simulink model "linear_bounded"  (R2017b)
settings: Solver=VariableStepAuto  StartTime=0.0  StopTime=1000  FixedStep=10e-3
settings Model: Creator=Mehmet  LastModifiedBy=Mehmet

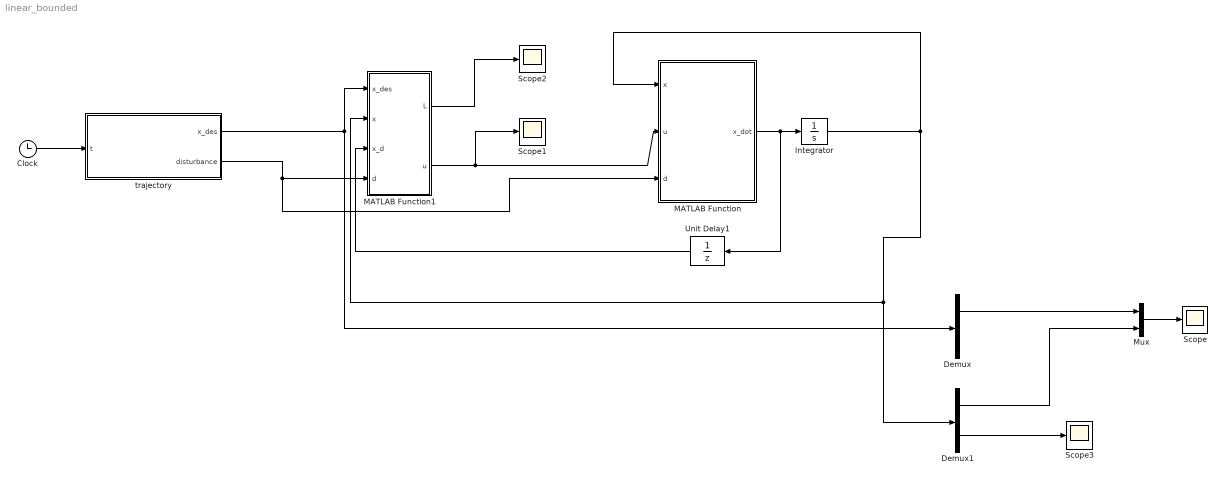
== system linear_bounded ==
  Clock : Clock
  Demux : Demux  Outputs=2
  Demux1 : Demux  Outputs=2
  Integrator : Integrator  InitialCondition=[1;-1]
  MATLAB Function : MATLAB Function  TreatAsAtomicUnit=on
  MATLAB Function1 : MATLAB Function  TreatAsAtomicUnit=on
  Mux : Mux  Inputs=2
  Scope{,1..3} (4 alike) : Scope
  Unit Delay1 : UnitDelay  SampleTime=-1
  trajectory : MATLAB Function  TreatAsAtomicUnit=on
  wires:
  Clock/1 -> trajectory/1(t)
  trajectory/1(x_des) -> MATLAB Function1/1(x_des), Demux/1
  Mux/1 -> Scope/1
  MATLAB Function/1(x_dot) -> Unit Delay1/1, Integrator/1
  Integrator/1 -> Demux1/1, MATLAB Function1/2(x), MATLAB Function/1(x)
  Unit Delay1/1 -> MATLAB Function1/3(x_d)
  trajectory/2(disturbance) -> MATLAB Function1/4(d), MATLAB Function/3(d)
  MATLAB Function1/2(u) -> Scope1/1, MATLAB Function/2(u)
  MATLAB Function1/1(L) -> Scope2/1
  Demux/1 -> Mux/1
  Demux1/1 -> Mux/2
  Demux1/2 -> Scope3/1

== matlab function linear_bounded/MATLAB Function1 ==
  data: L output; x_des input; u output; x input; x_d input; d input
function [L,u]= fcn(x_des,x,x_d,d)

K = 1;
Kp = 10;

e = (x_des(1) - x(1));
e_d = x_des(2) - x_d(1);

% u = x(2)*sin(x(1)) - K*x(2);

u = K*x(2)*(sin(x(1)) + e*x_des(1) - e^2) - K/x(2)*(e*x_des(2) + 10*x_des(1)*e);

L = 1/2*(e^2 + x(2)^2);

end

== matlab function linear_bounded/MATLAB Function ==
  data: x input; u input; x_dot output; d input
function x_dot = fcn(x,u,d)

q = zeros(2,1);

q(1) = x(1)*x(2) - 10*x(1);
q(2) = -x(1)^2*x(2) - x(2)*sin(x(1)) + u(1);

x_dot = q;

end

== matlab function linear_bounded/trajectory ==
  data: t input; x_des output; disturbance output
function [x_des,disturbance]= fcn(t)

A = 2;
B = 1;
f = 1;
w = 2*pi*f;

y = A*sin(w*t);
y_d = A*w*cos(w*t);

y = 5;
y_d = 0;


x_des = [y y_d]';

disturbance = B*cos(w*t)+1;
d = 0;
end
